simulink model "soc_dvbs2_fpga"  (R2025b)
settings: Solver=FixedStepDiscrete  StartTime=0.0  StopTime=0  RelTol=1e-3
InitFcn:
  | soc_dvbs2_init;
values from neighbouring files (symbols this model uses):
  Rsym = 4e6    (= 4000000)    [soc_dvbs2_init.m]
  soc_dvbs2_txPacketBits = [1 1 0 1 0 1 1 1 0 1 1 1 ... (2972 elements, 2972x1)]    [soc_dvbs2_txPacketBits.mat]
  syncWord = (dec2bin(hex2dec('AC')) - '0').'    [soc_dvbs2_init.m]
  txDataOut = txobj(frameBits(:))    [soc_dvbs2_init.m]
  txFiltCoeff = txobj.pTxFilterCoeff    [soc_dvbs2_init.m]
undefined symbols (not defined in the file or in its folder): Add, coefficientsLog, coefficientsSqrt1, coefficientsSqrt2, dataBits, designMultirateFIR, noisePow, NumBits1, NumBits2, seedsURNG1, seedsURNG2, Shift, Slope1, Slope2, soc_dvbs2_designFIRFilter, txDataOutS1, txDataOutS10, txDataOutS12, txDataOutS13, txDataOutS14, txDataOutS15, txDataOutS16, txDataOutS18, txDataOutS19, txDataOutS2, txDataOutS20, txDataOutS21, txDataOutS22, txDataOutS24, txDataOutS25, txDataOutS26, txDataOutS27, txDataOutS3, txDataOutS4, txDataOutS5, txDataOutS6, txDataOutS7, txDataOutS8, txDataOutS9
libraries: simulink x214, hdlsllib x211, dspsigops x22, dsphdlfiltering2 x8, dsphdlsigops2 x5, commseqgen3 x5, dsphdlmathfun2 x3, hwlogicconnlib x2, whdledac x2, commhdlcrc x2, whdlutilities x1, whdlmod x1
(part 8 of 12)

== system soc_dvbs2_fpga/DVBS2/DVBS2 TxRx/DVB-S2 HDL Receiver/Synchronizer and PL Header Decoder/Time Frequency and Coarse Phase Synchronizer/Fine Frequency Synchronizer/Modified L and R Algorithm/L and R Algorithm 18 point ==
  z : Inport
  zvalid : Inport  Port=2
  Add : Sum  Inputs=+++
  Compute R(m) for 1 to 6 : Subsystem  mask{m=1:6}
      mask prompts: m "m values for computing R(m):"
  Compute R(m) for 13 to 18 : Subsystem  mask{m=13:18}
      mask prompts: m "m values for computing R(m):"
  Compute R(m) for 7 to 12 : Subsystem  mask{m=7:12}
      mask prompts: m "m values for computing R(m):"
  Data Type Conversion : DataTypeConversion  OutDataTypeStr=fixdt(1,16,11)  SaturateOnIntegerOverflow=off  RndMeth=Floor
  Delay{1..6} (6 alike) : Delay
  dataIn : Outport
  wires:
  Data Type Conversion/1 -> Delay3/1
  Add/1 -> Delay6/1
  z/1 -> Data Type Conversion/1
  Delay3/1 -> Compute R(m) for 1 to 6/1(z), Compute R(m) for 13 to 18/1(z), Compute R(m) for 7 to 12/1(z)
  Delay2/1 -> Add/1
  Delay6/1 -> dataIn/1
  Delay5/1 -> Add/3
  Delay4/1 -> Add/2
  Delay1/1 -> Compute R(m) for 1 to 6/2(zvalid), Compute R(m) for 13 to 18/2(zvalid), Compute R(m) for 7 to 12/2(zvalid)
  Compute R(m) for 13 to 18/1(sum) -> Delay5/1
  Compute R(m) for 7 to 12/1(sum) -> Delay4/1
  Compute R(m) for 1 to 6/1(sum) -> Delay2/1
  zvalid/1 -> Delay1/1

== system soc_dvbs2_fpga/DVBS2/DVBS2 TxRx/DVB-S2 HDL Receiver/Synchronizer and PL Header Decoder/Time Frequency and Coarse Phase Synchronizer/Fine Frequency Synchronizer/Modified L and R Algorithm/Moving Average ==
  dataIn : Inport
  validIn : Inport  Port=2
  Add : Sum  Inputs=|++  OutDataTypeStr=Inherit: Inherit via back propagation
  Add1 : Sum  Inputs=|+-
  Data Type Duplicate : DataTypeDuplicate
  Data Type Conversion1 : DataTypeConversion  OutDataTypeStr=fixdt(1,53,36)  SaturateOnIntegerOverflow=off  RndMeth=Floor
  Delay : Delay  DelayLength=config.FFCAveragingLength  ShowEnablePort=on
      settings: InputPortMap=u0,e6
  Delay1 : Delay  DelayLength=1  ShowEnablePort=on
      settings: InputPortMap=u0,e6
  Delay2 : Delay
  Delay3 : Delay
  Delay{4..8} (5 alike) : Delay  DelayLength=1
  Gain : Gain  Gain=1/config.FFCAveragingLength  ParamDataTypeStr=fixdt(0,nextpow2(config.FFCAveragingLength),nextpow2(config.FFCAveragingLength))  OutDataTypeStr=Inherit: Same as input
  dataOut : Outport
  validOut : Outport  Port=2
  wires:
  Data Type Conversion1/1 -> Delay3/1
  Delay8/1 -> validOut/1
  Delay4/1 -> dataOut/1
  Gain/1 -> Add/1, Data Type Duplicate/1
  Delay7/1 -> Delay2/1
  Delay6/1 -> Add1/2
  Delay5/1 -> Add1/1
  Delay2/1 -> Delay1/2, Delay8/1
  Delay3/1 -> Gain/1
  validIn/1 -> Delay/2, Delay7/1
  Delay/1 -> Delay6/1
  Add1/1 -> Data Type Conversion1/1
  Add/1 -> Delay1/1, Delay4/1, Data Type Duplicate/2
  Delay1/1 -> Add/2
  dataIn/1 -> Delay/1, Delay5/1

== system soc_dvbs2_fpga/DVBS2/DVBS2 TxRx/DVB-S2 HDL Receiver/Synchronizer and PL Header Decoder/Time Frequency and Coarse Phase Synchronizer/Fine Gain Control/Reciprocal/Function Impl ==
  switch : Inport
  LUTAddr : Inport  Port=2
  Delay{6..8,10,15..16} (6 alike) : Delay
  Delay9 : Delay  DelayLength=1
  LUT1 : LookupNDDirect  NumberOfTableDimensions=1  Table=LUT(:,1)  DiagnosticForOutOfRangeInput=Error
  LUT2 : LookupNDDirect  NumberOfTableDimensions=1  Table=LUT(:,2)  DiagnosticForOutOfRangeInput=Error
  Multiport Switch : MultiPortSwitch  DataPortOrder=Zero-based contiguous  Inputs=2  zeroidx=on  SaturateOnIntegerOverflow=off  InputSameDT=off
  functionValues : Outport
  wires:
  LUTAddr/1 -> Delay7/1, Delay6/1
  Delay15/1 -> Multiport Switch/2
  Delay16/1 -> Multiport Switch/3
  Delay10/1 -> Multiport Switch/1
  Delay9/1 -> functionValues/1
  LUT2/1 -> Delay15/1
  LUT1/1 -> Delay16/1
  switch/1 -> Delay8/1
  Delay8/1 -> Delay10/1
  Delay7/1 -> LUT2/1
  Delay6/1 -> LUT1/1
  Multiport Switch/1 -> Delay9/1

== system soc_dvbs2_fpga/DVBS2/DVBS2 TxRx/DVB-S2 HDL Receiver/Synchronizer and PL Header Decoder/Time Frequency and Coarse Phase Synchronizer/Time and Coarse Frequency Synchronizer/Coarse Frequency Estimator/Direct Digital Synthesis ==
  v : Inport
  rst : Inport  Port=2
  Constant : Constant  Value=true  SampleTime=-1
  Data Type Conversion : DataTypeConversion  OutDataTypeStr=fixdt(1,21,21)  SaturateOnIntegerOverflow=off  RndMeth=Floor
  Data Type Conversion1 : DataTypeConversion  OutDataTypeStr=fixdt(1,21,0)  ConvertRealWorld=Stored Integer (SI)  SaturateOnIntegerOverflow=off  RndMeth=Floor
  Delay1 : Delay
  Delay14 : Delay
  Delay2 : Delay  DelayLength=1  InitialCondition=0
  Gain : Gain  Gain=1/config.SamplesPerSymbol  ParamDataTypeStr=fixdt(0,2,2)  OutDataTypeStr=Inherit: Same as input
  NCO HDL Optimized : dsphdlsigops2/NCO  PhaseIncrementSource=Input port  PhaseIncrement=100  PhaseOffsetSource=Property  PhaseOffset=0  DitherSource=None  NumDitherBits=11  SamplesPerFrame=1  LUTCompress=off  ResetAction=on  Waveform=Complex exponential  PhasePort=off  SimulateUsing=Code generation  AccumulatorWL=21  PhaseQuantization=on  NumQuantizerAccumulatorBits=14  OutputDataType=Binary point scaling  OutputWL=16  OutputFL=14
  Repeat : dspsigops/Repeat  FactorSource=Dialog parameter  N=config.SamplesPerSymbol  Nmax=16  RateOptions=Allow multirate processing  ic=0  mode=Unused parameter value
  Repeat1 : dspsigops/Repeat  FactorSource=Dialog parameter  N=config.SamplesPerSymbol  Nmax=16  RateOptions=Allow multirate processing  ic=0  mode=Unused parameter value
  Terminator : Terminator
  complexEst : Outport
  normalizedEst : Outport  Port=2
  wires:
  Repeat1/1 -> NCO HDL Optimized/2
  rst/1 -> Repeat1/1
  Data Type Conversion/1 -> normalizedEst/1, Data Type Conversion1/1
  Repeat/1 -> NCO HDL Optimized/1
  Constant/1 -> NCO HDL Optimized/3
  Data Type Conversion1/1 -> Repeat/1
  Delay2/1 -> complexEst/1
  Delay1/1 -> Data Type Conversion/1
  Delay14/1 -> Gain/1
  NCO HDL Optimized/1 -> Delay2/1
  v/1 -> Delay14/1
  NCO HDL Optimized/2 -> Terminator/1
  Gain/1 -> Delay1/1

== system soc_dvbs2_fpga/DVBS2/DVBS2 TxRx/DVB-S2 HDL Receiver/Synchronizer and PL Header Decoder/Time Frequency and Coarse Phase Synchronizer/Time and Coarse Frequency Synchronizer/Coarse Frequency Estimator/Frequency Error Detector ==
  dataIn : Inport
  pilotIdx : Inport  Port=2
  pilotValid : Inport  Port=3
  Compare To Constant1 : simulink/Logic and Bit Operations/Compare To Constant  relop=<=  const=config.PilotMaxIdx - 2  OutDataTypeStr=boolean
  Compare To Constant2 : simulink/Logic and Bit Operations/Compare To Constant  relop=>=  const=config.PilotMinIdx + 2  OutDataTypeStr=boolean
  Complex Multiplier : Subsystem  VariantControl=Use 3 multipliers and 5 adders
      mask Display: disp(['Complex Multiplier' newline 'Latency = 8']);
  Complex to Real-Imag : ComplexToRealImag  Output=Imag
  Delay{,1..11,16..19,24} (17 alike) : Delay
  Delay12 : Delay  DelayLength=1
  Delay13 : Delay  DelayLength=1
  Delay14 : Delay  DelayLength=1
  Delay15 : Delay  DelayLength=8
  Gain : Gain  Gain=conj(config.Pilot)  OutDataTypeStr=Inherit: Same as input
      mask init:
      | Simulink.suppressDiagnostic(gcb, 'SimulinkFixedPoint:util:fxpParameterPrecisionLoss');
  Gain1 : Gain  Gain=config.Pilot  OutDataTypeStr=Inherit: Same as input
      mask init:
      | Simulink.suppressDiagnostic(gcb, 'SimulinkFixedPoint:util:fxpParameterPrecisionLoss');
  Logical Operator : Logic  Inputs=3  AllPortsSameDT=off  OutDataTypeStr=boolean
  Math Function : Math  Operator=conj
  Unit Delay Enabled Synchronous : hdlsllib/Discrete/Unit Delay Enabled Synchronous  InitialCondition=0.0  SampleTime=-1
  e : Outport
  wires:
  Delay19/1 -> Complex Multiplier/1(In1)
  Delay17/1 -> Complex Multiplier/2(In2)
  Delay16/1 -> Delay15/1
  Delay14/1 -> e/1
  Complex Multiplier/1(Out1) -> Delay10/1
  Delay18/1 -> Logical Operator/2
  Compare To Constant1/1 -> Delay18/1
  Logical Operator/1 -> Delay8/1
  Gain1/1 -> Delay6/1
  Gain/1 -> Delay4/1
  Delay15/1 -> Delay11/1
  Delay7/1 -> Delay17/1
  Delay5/1 -> Delay19/1
  Delay13/1 -> Unit Delay Enabled Synchronous/2
  Delay12/1 -> Unit Delay Enabled Synchronous/1
  Delay11/1 -> Delay13/1
  Delay10/1 -> Complex to Real-Imag/1
  Delay9/1 -> Delay16/1
  Delay8/1 -> Delay9/1
  Delay6/1 -> Delay7/1
  Delay4/1 -> Delay5/1
  Delay3/1 -> Logical Operator/3
  Delay2/1 -> Logical Operator/1
  Delay1/1 -> Gain1/1
  Delay24/1 -> Gain/1
  Complex to Real-Imag/1 -> Delay12/1
  pilotValid/1 -> Delay3/1
  Compare To Constant2/1 -> Delay2/1
  pilotIdx/1 -> Compare To Constant2/1, Compare To Constant1/1
  Unit Delay Enabled Synchronous/1 -> Delay14/1
  Math Function/1 -> Delay1/1
  dataIn/1 -> Delay/1, Delay24/1
  Delay/1 -> Math Function/1

== system soc_dvbs2_fpga/DVBS2/DVBS2 TxRx/DVB-S2 HDL Receiver/Synchronizer and PL Header Decoder/Time Frequency and Coarse Phase Synchronizer/Time and Coarse Frequency Synchronizer/Coarse Frequency Estimator/Loop Filter ==
  e : Inport
  rst : Inport  Port=2
  En : Inport  Port=3
  Add : Sum  Inputs=|++  OutDataTypeStr=Inherit: Same as first input
  Delay{,1..3} (4 alike) : Delay  DelayLength=1
  Delay14 : Delay
  Integrator Gain : Gain  Gain=fi(config.CFCLoopFilterIntegGain/(2*pi),0,16)  ParamDataTypeStr=Inherit: Inherit from 'Gain'  OutDataTypeStr=Inherit: Same as input
  Unit Delay Enabled Resettable Synchronous : hdlsllib/Discrete/Unit Delay Enabled Resettable Synchronous  InitialCondition=0.0  SampleTime=-1
  v : Outport
  rstOut : Outport  Port=2
  wires:
  Delay/1 -> Delay3/1
  Delay3/1 -> rstOut/1
  rst/1 -> Unit Delay Enabled Resettable Synchronous/3, Delay/1
  Add/1 -> Unit Delay Enabled Resettable Synchronous/1
  En/1 -> Unit Delay Enabled Resettable Synchronous/2
  Unit Delay Enabled Resettable Synchronous/1 -> Delay2/1, Add/2
  Delay1/1 -> Add/1
  Delay2/1 -> v/1
  Delay14/1 -> Integrator Gain/1
  e/1 -> Delay14/1
  Integrator Gain/1 -> Delay1/1

== system soc_dvbs2_fpga/DVBS2/DVBS2 TxRx/DVB-S2 HDL Receiver/Synchronizer and PL Header Decoder/Time Frequency and Coarse Phase Synchronizer/Time and Coarse Frequency Synchronizer/Coarse Frequency Estimator/Pilot Blks Counter ==
  pilotIdx : Inport
  pilotValid : Inport  Port=2
  rst : Inport  Port=3
  Compare To Constant : simulink/Logic and Bit Operations/Compare To Constant  relop===  const=config.PilotMinIdx  OutDataTypeStr=boolean
  HDL Counter : hdlsllib/Sources/HDL Counter  CountType=Free running  CountInit=0  CountStep=1  CountMax=25  CountFromType=Initial value  CountFrom=0  CountResetPort=on  CountLoadPort=off  CountEnbPort=on  CountDirPort=off  CountHitOutputPort=off  CountDataType=Unsigned  CountWordLen=16  CountFracLen=0  CountSampTime=1
  Logical Operator : Logic  AllPortsSameDT=off  OutDataTypeStr=boolean
  pilotBlkCount : Outport
  wires:
  rst/1 -> HDL Counter/1
  HDL Counter/1 -> pilotBlkCount/1
  pilotIdx/1 -> Compare To Constant/1
  pilotValid/1 -> Logical Operator/2
  Compare To Constant/1 -> Logical Operator/1
  Logical Operator/1 -> HDL Counter/2

== system soc_dvbs2_fpga/DVBS2/DVBS2 TxRx/DVB-S2 HDL Receiver/Synchronizer and PL Header Decoder/Time Frequency and Coarse Phase Synchronizer/Time and Coarse Frequency Synchronizer/Frame Synchronizer/Correlator ==
  note: Differential Detection
  note: Compute Energy
  dataIn : Inport
  validIn : Inport  Port=2
  Add4 : Sum
  Complex to Real-Imag : ComplexToRealImag  Output=Real
  Data Type Conversion : DataTypeConversion  OutDataTypeStr=fixdt(1,17,14)  SaturateOnIntegerOverflow=off  RndMeth=Floor
  Delay{,9..10,12} (4 alike) : Delay  DelayLength=1
  Delay{1..2,4..8,11,13..25} (21 alike) : Delay
  Delay3 : Delay  DelayLength=70-32
  Gain : Gain  Gain=fi(config.refSOFE,0,16,16)  OutDataTypeStr=fixdt(1,32,30)
  Gain1 : Gain  Gain=fi(config.refPLSCE,0,16,16)  OutDataTypeStr=fixdt(1,32,30)
  Math Function : Math  Operator=conj
  Math Function1 : Math  Operator=conj
  Moving Sum : Subsystem
  PLSC Correlator : Subsystem  mask{coefs=config.refPLSC, shareFactor=4}
      mask prompts: coefs "Coefficients:"; shareFactor "Number of cycles:"
      mask init:
      | ob                         = dsphdl.FIRFilter('Numerator',coefs);
      | directFormLatency          = getLatency(ob);
      | 
      | ob                         = dsphdl.FIRFilter('Numerator',coefs,...
      |                                               'FilterStructure','Partly Serial Systolic',...
      |                                               'NumCycles',shareFactor);
      | partlySerialLatency        = getLatency(ob);
      | partlySerialExtraDelay     = 4 - mod(partlySerialLatency,4);
      | 
      | adjustDelay                = directFormLatency - ...
      |                             (partlySerialLatency+partlySerialExtraDelay)/shareFactor;
  Product : Product  OutDataTypeStr=Inherit: Same as first input
  Product1 : Product  OutDataTypeStr=Inherit: Same as first input
  SOF Correlator : Subsystem  mask{coefs=config.refSOF, shareFactor=4}
      mask prompts: coefs "Coefficients:"; shareFactor "Number of cycles:"
      mask init: same as soc_dvbs2_fpga/DVBS2/DVBS2 TxRx/DVB-S2 HDL Receiver/Synchronizer and PL Header Decoder/Time Frequency and Coarse Phase Synchronizer/Time and Coarse Frequency Synchronizer/Frame Synchronizer/Correlator/PLSC Correlator
  SOFCorrOut : Outport
  PLSCCorrOut : Outport  Port=2
  threshold : Outport  Port=3
  wires:
  SOF Correlator/1(dataOut) -> Delay3/1
  Delay25/1 -> Moving Sum/3(validIn)
  Delay11/1 -> Delay25/1
  Delay24/1 -> Delay4/1
  Delay23/1 -> Delay5/1
  Delay22/1 -> Delay6/1
  Delay21/1 -> Delay11/1
  Delay20/1 -> Complex to Real-Imag/1
  Delay19/1 -> Product1/1
  Delay18/1 -> Product1/2
  Delay17/1 -> Delay21/1
  Delay16/1 -> Gain1/1
  Delay15/1 -> Gain/1
  Delay14/1 -> Moving Sum/1(scaled1)
  Delay13/1 -> Moving Sum/2(scaled2)
  dataIn/1 -> Delay1/1, Delay19/1, Math Function1/1
  Math Function1/1 -> Delay18/1
  Complex to Real-Imag/1 -> Delay16/1, Delay15/1
  Add4/1 -> Delay12/1
  Delay12/1 -> Data Type Conversion/1
  Product1/1 -> Delay20/1
  Gain/1 -> Delay14/1
  validIn/1 -> Delay17/1, Delay2/1
  Gain1/1 -> Delay13/1
  Moving Sum/1(E1) -> Add4/1
  Moving Sum/2(E2) -> Add4/2
  PLSC Correlator/1(dataOut) -> Delay10/1
  Delay3/1 -> Delay9/1
  Product/1 -> Delay7/1
  Math Function/1 -> Delay24/1
  Delay/1 -> Delay23/1
  Delay1/1 -> Math Function/1, Delay/1
  Delay2/1 -> Delay22/1
  Delay4/1 -> Product/1
  Delay5/1 -> Product/2
  Delay6/1 -> Delay8/1
  Delay8/1 -> SOF Correlator/2(validIn), PLSC Correlator/2(validIn)
  Delay7/1 -> SOF Correlator/1(dataIn), PLSC Correlator/1(dataIn)
  Delay10/1 -> PLSCCorrOut/1
  Delay9/1 -> SOFCorrOut/1
  Data Type Conversion/1 -> threshold/1

== system soc_dvbs2_fpga/DVBS2/DVBS2 TxRx/DVB-S2 HDL Receiver/Synchronizer and PL Header Decoder/Time Frequency and Coarse Phase Synchronizer/Time and Coarse Frequency Synchronizer/Frame Synchronizer/Pilot and Sync Pulse Indicator ==
  note: Compute Energy
  note: Compute Energy
  SOFCorrDelayed : Inport
  PLSCCorr : Inport  Port=2
  threshold : Inport  Port=3
  Bus Creator : BusCreator  Inputs=3
  Complex to Real-Imag : ComplexToRealImag  Output=Real
  Complex to Real-Imag1 : ComplexToRealImag  Output=Real
  Corr Add : Sum
  Corr Subtract : Sum  Inputs=+-
  Delay{1..10,15..16,19..21,24..26} (18 alike) : Delay  DelayLength=1
  Delay{11..14,17..18,22..23} (8 alike) : Delay
  Logical Operator : Logic  Operator=OR  AllPortsSameDT=off  OutDataTypeStr=boolean
  Math Function : Math  Operator=conj
  Math Function1 : Math  Operator=conj
  No HDL Correlation Value : Subsystem
  Product : Product  OutDataTypeStr=fixdt(1,18,15)
  Product1 : Product  OutDataTypeStr=fixdt(1,18,15)
  Relational Operator : RelationalOperator  Operator=>  OutDataTypeStr=boolean  RndMeth=Simplest  InputSameDT=off
  Relational Operator1 : RelationalOperator  Operator=>  OutDataTypeStr=boolean  RndMeth=Simplest  InputSameDT=off
  Threshold Scaling : Gain  Gain=config.Threshold  OutDataTypeStr=Inherit: Same as input
      mask init:
      | Simulink.suppressDiagnostic(gcb, 'SimulinkFixedPoint:util:fxpParameterPrecisionLoss');
  ThresholdLimiter : MATLAB Function  TreatAsAtomicUnit=on
  hasPilots : Outport
  thresholdExceeded : Outport  Port=2
  VisualizeCorrelationSignals : Outport  Port=3
  wires:
  Delay9/1 -> hasPilots/1, No HDL Correlation Value/2(In1)
  Complex to Real-Imag1/1 -> Delay1/1
  Complex to Real-Imag/1 -> Delay6/1
  Delay24/1 -> Delay22/1
  Delay12/1 -> Complex to Real-Imag1/1
  Delay19/1 -> Math Function1/1
  Delay18/1 -> Product1/2
  Delay20/1 -> Delay17/1
  Delay17/1 -> Product1/1
  Corr Subtract/1 -> Delay20/1, Delay19/1
  Product1/1 -> Delay12/1
  Math Function1/1 -> Delay18/1
  ThresholdLimiter/1(y) -> Delay26/1
  Delay10/1 -> thresholdExceeded/1
  Delay25/1 -> ThresholdLimiter/1(x)
  Delay23/1 -> Delay25/1
  Threshold Scaling/1 -> Delay23/1
  Delay22/1 -> Threshold Scaling/1
  Delay21/1 -> Delay24/1
  threshold/1 -> Delay21/1
  PLSCCorr/1 -> Delay5/1, Delay3/1
  SOFCorrDelayed/1 -> Delay4/1, Delay2/1
  Delay1/1 -> Delay8/1
  Delay6/1 -> Delay7/1
  Product/1 -> Delay11/1
  Delay16/1 -> Delay13/1
  Delay15/1 -> Math Function/1
  Delay14/1 -> Product/2
  Delay11/1 -> Complex to Real-Imag/1
  Math Function/1 -> Delay14/1
  Corr Add/1 -> Delay16/1, Delay15/1
  Delay13/1 -> Product/1
  Delay5/1 -> Corr Subtract/2
  Delay4/1 -> Corr Subtract/1
  Delay3/1 -> Corr Add/2
  Delay2/1 -> Corr Add/1
  Relational Operator/1 -> Logical Operator/1, Delay9/1
  Logical Operator/1 -> Delay10/1
  Relational Operator1/1 -> Logical Operator/2
  Delay7/1 -> Bus Creator/1, No HDL Correlation Value/1(PeakValueWithPilots), Relational Operator/1  "PeakValueWithPilots"
  Delay26/1 -> Relational Operator/2, Bus Creator/3, Relational Operator1/2  "Threshold"
  Delay8/1 -> Bus Creator/2, No HDL Correlation Value/3(PeakValueWithoutPilots), Relational Operator1/1  "PeakValueWithoutPilots"
  Bus Creator/1 -> VisualizeCorrelationSignals/1  "VisualizeCorrelationSignals"

== system soc_dvbs2_fpga/DVBS2/DVBS2 TxRx/DVB-S2 HDL Receiver/Synchronizer and PL Header Decoder/Time Frequency and Coarse Phase Synchronizer/Time and Coarse Frequency Synchronizer/PL Data Descrambler and Pilot Valid Indicator/PL Data Descrambler ==
  reset : Inport
  inputCount : Inport  Port=2
  validIn : Inport  Port=3
  dataIn : Inport  Port=4
  Compare To Constant : simulink/Logic and Bit Operations/Compare To Constant  relop=<=  const=config.PLSCLength - 1  OutDataTypeStr=boolean
  Delay1 : Delay  DelayLength=7
  Delay{2..8,10..12,22..23} (12 alike) : Delay  DelayLength=1
  Delay{13..21} (9 alike) : Delay
  Delay9 : Delay  DelayLength=7
  Math Function : Math  Operator=conj
  PL Scramble Sequence Mapper LUT : Lookup_n-D  NumberOfTableDimensions=1  LookupTableObject=''  BreakpointsSpecification=Even spacing  BreakpointsForDimension1=[-5:5]  BreakpointsForDimension1FirstPoint=0  BreakpointsForDimension2FirstPoint=10  BreakpointsForDimension2Spacing=12  IndexSearchMethod=Evenly spaced points  Table=[1;1i;-1;-1i]  TableDataTypeStr=fixdt(1,2,0)  InterpMethod=Flat  DiagnosticForOutOfRangeInput=Error  InternalRulePriority=Speed  OutDataTypeStr=fixdt(1,2,0)  RndMeth=Simplest
  PL Scrambler Gold Sequence Generator : Subsystem  mask{n=0}
      mask prompts: n "Index of Gold Sequence :"
  Product : Product  OutDataTypeStr=Inherit: Same as first input
  Switch : Switch  Criteria=u2 ~= 0  SaturateOnIntegerOverflow=off  InputSameDT=off
  dataOut : Outport
  validOut : Outport  Port=2
  wires:
  Delay12/1 -> Delay13/1
  Delay23/1 -> validOut/1
  Delay22/1 -> dataOut/1
  Delay21/1 -> Delay23/1
  Delay20/1 -> Switch/3
  Delay19/1 -> Switch/2
  Delay18/1 -> Switch/1
  Delay17/1 -> Delay21/1
  Delay16/1 -> Product/2
  Delay15/1 -> Product/1
  Delay14/1 -> Delay19/1
  Delay13/1 -> Delay18/1
  Delay11/1 -> Compare To Constant/1
  Delay10/1 -> Delay15/1
  Delay8/1 -> Delay17/1
  Delay7/1 -> Math Function/1
  Delay6/1 -> Delay12/1
  Delay5/1 -> Delay8/1
  Delay4/1 -> Delay10/1
  Delay3/1 -> Delay11/1
  Delay2/1 -> PL Scramble Sequence Mapper LUT/1
  Delay1/1 -> Delay3/1
  Delay9/1 -> Delay6/1, Delay4/1
  validIn/1 -> PL Scrambler Gold Sequence Generator/2(validIn)
  reset/1 -> PL Scrambler Gold Sequence Generator/1(reset)
  PL Scrambler Gold Sequence Generator/2(validOut) -> Delay5/1
  Switch/1 -> Delay22/1
  Product/1 -> Delay20/1
  PL Scramble Sequence Mapper LUT/1 -> Delay7/1
  dataIn/1 -> Delay9/1
  Math Function/1 -> Delay16/1
  inputCount/1 -> Delay1/1
  Compare To Constant/1 -> Delay14/1
  PL Scrambler Gold Sequence Generator/1(dataOut) -> Delay2/1

== system soc_dvbs2_fpga/DVBS2/DVBS2 TxRx/DVB-S2 HDL Receiver/Synchronizer and PL Header Decoder/Time Frequency and Coarse Phase Synchronizer/Time and Coarse Frequency Synchronizer/PL Data Descrambler and Pilot Valid Indicator/Pilot Valid Indicator ==
  note: Hold pilotEnable signal
  note: Hold pilotsEnable signal after endOfPLSC
  pilotEnable : Inport
  validIn : Inport  Port=2
  endOfSOFIn : Inport  Port=3
  endOfPLSC : Inport  Port=4
  Compare To Constant2 : simulink/Logic and Bit Operations/Compare To Constant  relop=>=  const=config.PilotMinIdx  OutDataTypeStr=boolean
  Compare To Constant3 : simulink/Logic and Bit Operations/Compare To Constant  relop=<=  const=config.PilotMaxIdx  OutDataTypeStr=boolean
  Delay{1..4} (4 alike) : Delay  DelayLength=config.SOFLength
  Delay{5..14,19} (11 alike) : Delay  DelayLength=1
  Delay15 : Delay
  Delay16 : Delay
  Delay17 : Delay
  Logical Operator1 : Logic  Inputs=3  AllPortsSameDT=off  OutDataTypeStr=boolean
  Logical Operator2 : Logic  AllPortsSameDT=off  OutDataTypeStr=boolean
  Logical Operator3 : Logic  AllPortsSameDT=off  OutDataTypeStr=boolean
  PilotIdx Counter : hdlsllib/Sources/HDL Counter  CountType=Count limited  CountInit=0  CountStep=1  CountMax=config.PilotMaxIdx  CountFromType=Initial value  CountFrom=0  CountResetPort=on  CountLoadPort=off  CountEnbPort=on  CountDirPort=off  CountHitOutputPort=off  CountDataType=Unsigned  CountWordLen=nextpow2(config.PilotMaxIdx)  CountFracLen=0  CountSampTime=1
  Unit Delay Enabled Resettable Synchronous : hdlsllib/Discrete/Unit Delay Enabled Resettable Synchronous  InitialCondition=0.0  SampleTime=-1
  Unit Delay Enabled Resettable Synchronous1 : hdlsllib/Discrete/Unit Delay Enabled Resettable Synchronous  InitialCondition=0.0  SampleTime=-1
  pilotValid : Outport
  pilotIdx : Outport  Port=2
  endOfSOF : Outport  Port=3
  wires:
  Delay17/1 -> endOfSOF/1
  Delay16/1 -> pilotValid/1
  Delay15/1 -> pilotIdx/1
  Delay14/1 -> Delay17/1
  Delay13/1 -> Logical Operator1/3
  Delay12/1 -> Logical Operator1/2
  Delay11/1 -> Logical Operator1/1
  Delay10/1 -> Delay15/1
  Delay9/1 -> Delay14/1
  Delay8/1 -> Delay13/1
  Delay7/1 -> Logical Operator3/2
  Delay6/1 -> Compare To Constant3/1
  Delay5/1 -> Compare To Constant2/1
  Delay19/1 -> Delay10/1
  Logical Operator3/1 -> Delay12/1
  Unit Delay Enabled Resettable Synchronous/1 -> Logical Operator2/2
  Unit Delay Enabled Resettable Synchronous1/1 -> Delay8/1
  Delay2/1 -> Delay9/1, Unit Delay Enabled Resettable Synchronous/2
  Delay1/1 -> Unit Delay Enabled Resettable Synchronous/1
  Delay4/1 -> Delay7/1, PilotIdx Counter/2
  Delay3/1 -> Logical Operator2/1, PilotIdx Counter/1
  endOfSOFIn/1 -> Delay2/1, Unit Delay Enabled Resettable Synchronous/3, Unit Delay Enabled Resettable Synchronous1/3
  pilotEnable/1 -> Delay1/1
  Logical Operator1/1 -> Delay16/1
  Logical Operator2/1 -> Unit Delay Enabled Resettable Synchronous1/2, Unit Delay Enabled Resettable Synchronous1/1
  validIn/1 -> Delay4/1
  Compare To Constant2/1 -> Delay11/1
  PilotIdx Counter/1 -> Delay19/1, Delay5/1, Delay6/1
  endOfPLSC/1 -> Delay3/1
  Compare To Constant3/1 -> Logical Operator3/1

== system soc_dvbs2_fpga/DVBS2/DVBS2 TxRx/DVB-S2 HDL Receiver/Synchronizer and PL Header Decoder/Time Frequency and Coarse Phase Synchronizer/Time and Coarse Frequency Synchronizer/Symbol Synchronizer/Gardner TED ==
  data : Inport
  strobe : Inport  Port=2
  Constant : Constant  Value=0  OutDataTypeStr=Inherit: Inherit via back propagation  SampleTime=-1
  Delay10 : Delay  DelayLength=4
  GTED : Subsystem
  Switch : Switch  Criteria=u2 ~= 0  InputSameDT=off
  e : Outport  VectorParamsAs1DForOutWhenUnconnected=off
  wires:
  Delay10/1 -> Switch/2
  GTED/1(Out1) -> Switch/1
  data/1 -> GTED/1(In1)
  strobe/1 -> Delay10/1
  Switch/1 -> e/1
  Constant/1 -> Switch/3

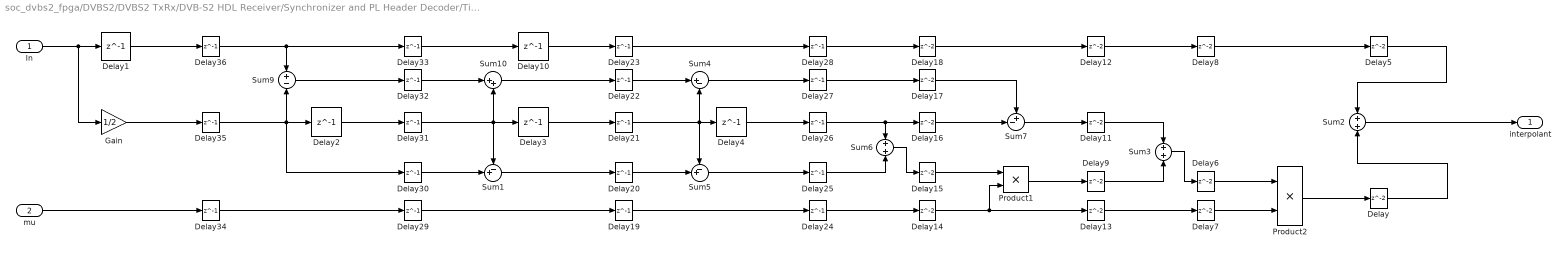
== system soc_dvbs2_fpga/DVBS2/DVBS2 TxRx/DVB-S2 HDL Receiver/Synchronizer and PL Header Decoder/Time Frequency and Coarse Phase Synchronizer/Time and Coarse Frequency Synchronizer/Symbol Synchronizer/Interpolation Filter ==
  In : Inport
  mu : Inport  Port=2
  Delay{,5..9,11..18} (14 alike) : Delay
  Delay{1..4,10} (5 alike) : Delay  DelayLength=1  InitialCondition=0
  Delay{19..36} (18 alike) : Delay  DelayLength=1
  Gain : Gain  Gain=1/2  ParamDataTypeStr=fixdt(0,1,1)  OutDataTypeStr=Inherit: Same as input
  Product1 : Product  RndMeth=Zero  OutDataTypeStr=Inherit: Same as first input
  Product2 : Product  RndMeth=Zero  OutDataTypeStr=Inherit: Same as first input
  Sum1 : Sum  Inputs=-+|
  Sum10 : Sum  Inputs=|++
  Sum2 : Sum  Inputs=+|+
  Sum3 : Sum  Inputs=+|+  OutDataTypeStr=Inherit: Same as first input
  Sum4 : Sum  Inputs=|+-
  Sum5 : Sum  Inputs=-+|
  Sum6 : Sum  Inputs=+|+  SaturateOnIntegerOverflow=on  OutDataTypeStr=Inherit: Same as first input
  Sum7 : Sum  Inputs=+-|  OutDataTypeStr=Inherit: Same as first input
  Sum9 : Sum  Inputs=+-
  interpolant : Outport
  wires:
  Delay36/1 -> Sum9/1, Delay33/1
  Delay35/1 -> Sum9/2, Delay2/1, Delay30/1
  Delay34/1 -> Delay29/1
  Delay33/1 -> Delay10/1
  Delay32/1 -> Sum10/1
  Delay31/1 -> Delay3/1, Sum10/2, Sum1/1
  Delay30/1 -> Sum1/2
  Delay29/1 -> Delay19/1
  Delay23/1 -> Delay28/1
  Delay22/1 -> Sum4/1
  Delay21/1 -> Delay4/1, Sum5/1, Sum4/2
  Delay20/1 -> Sum5/2
  Delay19/1 -> Delay24/1
  Delay25/1 -> Sum6/2
  Delay28/1 -> Delay18/1
  Delay27/1 -> Delay17/1
  Delay26/1 -> Sum6/1, Delay16/1
  Sum6/1 -> Delay15/1
  Delay24/1 -> Delay14/1
  Delay10/1 -> Delay23/1
  Sum4/1 -> Delay27/1
  Delay4/1 -> Delay26/1
  Sum5/1 -> Delay25/1
  mu/1 -> Delay34/1
  Delay18/1 -> Delay12/1
  Delay17/1 -> Sum7/1
  Delay16/1 -> Sum7/2
  Delay15/1 -> Product1/1
  Delay14/1 -> Product1/2, Delay13/1
  Delay13/1 -> Delay7/1
  Delay12/1 -> Delay8/1
  Delay11/1 -> Sum3/1
  Delay9/1 -> Sum3/2
  Delay8/1 -> Delay5/1
  Delay7/1 -> Product2/2
  Delay6/1 -> Product2/1
  Delay5/1 -> Sum2/1
  Delay/1 -> Sum2/2
  Gain/1 -> Delay35/1
  Delay1/1 -> Delay36/1
  Delay2/1 -> Delay31/1
  Sum10/1 -> Delay22/1
  Delay3/1 -> Delay21/1
  Sum1/1 -> Delay20/1
  Sum3/1 -> Delay6/1
  Product2/1 -> Delay/1
  Product1/1 -> Delay9/1
  Sum7/1 -> Delay11/1
  Sum2/1 -> interpolant/1
  In/1 -> Gain/1, Delay1/1
  Sum9/1 -> Delay32/1

== system soc_dvbs2_fpga/DVBS2/DVBS2 TxRx/DVB-S2 HDL Receiver/Synchronizer and PL Header Decoder/Time Frequency and Coarse Phase Synchronizer/Time and Coarse Frequency Synchronizer/Symbol Synchronizer/Loop Filter ==
  note: Proportional-Plus-Integrator Loop Filter,
      | Infinite DC Response to guarantee convergence
  e : Inport
  Add : Sum
  Add2 : Sum  Inputs=|++  OutDataTypeStr=Inherit: Same as first input
  Data Type Conversion17 : DataTypeConversion  OutDataTypeStr=fixdt(1,11,10)  SaturateOnIntegerOverflow=off  RndMeth=Floor
  Delay : Delay  DelayLength=1
  Delay1 : Delay  DelayLength=1  InitialCondition=0
  Delay2 : Delay  InitialCondition=0
  Delay3 : Delay  InitialCondition=0
  Delay4 : Delay  DelayLength=1  InitialCondition=0
  Delay5 : Delay  InitialCondition=0
  Delay6 : Delay  DelayLength=1
  K1 : Gain  Gain=fi(config.SSLoopFilterPropGain,1,24,24)  ParamDataTypeStr=Inherit: Inherit from 'Gain'  OutDataTypeStr=Inherit: Same as input
  K2 : Gain  Gain=fi(config.SSLoopFilterIntegGain,1,24,24)  ParamDataTypeStr=Inherit: Inherit from 'Gain'  OutDataTypeStr=Inherit: Same as input
  v : Outport
  wires:
  Delay6/1 -> Add2/1
  K1/1 -> Delay3/1
  Add2/1 -> Delay4/1, Delay/1
  K2/1 -> Delay5/1
  Data Type Conversion17/1 -> v/1
  Delay2/1 -> K2/1, K1/1
  Delay4/1 -> Add/2
  Delay1/1 -> Add/1
  Add/1 -> Data Type Conversion17/1
  e/1 -> Delay2/1
  Delay3/1 -> Delay1/1
  Delay5/1 -> Delay6/1
  Delay/1 -> Add2/2

== system soc_dvbs2_fpga/DVBS2/DVBS2 TxRx/DVB-S2 HDL Receiver/Synchronizer and PL Header Decoder/Time Frequency and Coarse Phase Synchronizer/Time and Coarse Frequency Synchronizer/Symbol Synchronizer/Rate Handle ==
  dataIn : Inport
  strobe : Inport  Port=2
  validIn : Inport  Port=3
  Compare To Constant : simulink/Logic and Bit Operations/Compare To Constant  relop===  const=config.SamplesPerSymbol - 1  OutDataTypeStr=boolean
  Downsample : DownSample  N=config.SamplesPerSymbol  RateOptions=Allow multirate processing
  Downsample1 : DownSample  N=config.SamplesPerSymbol  RateOptions=Allow multirate processing
  FIFO : Subsystem
  HDL Counter : hdlsllib/Sources/HDL Counter  CountType=Count limited  CountInit=0  CountStep=1  CountMax=config.SamplesPerSymbol - 1  CountFromType=Initial value  CountFrom=0  CountResetPort=off  CountLoadPort=off  CountEnbPort=on  CountDirPort=off  CountHitOutputPort=off  CountDataType=Unsigned  CountWordLen=nextpow2(config.SamplesPerSymbol - 1)  CountFracLen=0  CountSampTime=1
  Logical Operator : Logic  AllPortsSameDT=off  OutDataTypeStr=boolean
  Unit Delay Enabled Synchronous : hdlsllib/Discrete/Unit Delay Enabled Synchronous  InitialCondition=0.0  SampleTime=-1
  monostable : MATLAB Function  TreatAsAtomicUnit=on  mask{nClocks=config.SamplesPerSymbol}
      mask prompts: nClocks "Number of Clocks:"
  dataOut : Outport
  validOut : Outport  Port=2
  wires:
  Unit Delay Enabled Synchronous/1 -> Downsample/1
  monostable/1(out) -> Downsample1/1
  FIFO/2(outValid) -> monostable/1(trigger), Unit Delay Enabled Synchronous/2
  FIFO/1(out) -> Unit Delay Enabled Synchronous/1
  Logical Operator/1 -> FIFO/3(pop)
  strobe/1 -> FIFO/2(push)
  dataIn/1 -> FIFO/1(data)
  validIn/1 -> Logical Operator/1, HDL Counter/1
  Downsample/1 -> dataOut/1
  Downsample1/1 -> validOut/1
  HDL Counter/1 -> Compare To Constant/1
  Compare To Constant/1 -> Logical Operator/2

== system soc_dvbs2_fpga/DVBS2/DVBS2 TxRx/DVB-S2 HDL Receiver/Demod Deinterleave and FECDecode/DVBS2 HDL Deinterleaver/RAM Address Generator/Generate and Add Read Base Address/No HDL Read Address Debug Scope/Wrap Address ==
  u : Inport
  Add : Sum  Inputs=+-  OutDataTypeStr=Inherit: Same as first input
  Compare To Constant : simulink/Logic and Bit Operations/Compare To Constant  relop=>=  const=ConfigRx.RAMCapacity  OutDataTypeStr=boolean
  Constant : Constant  Value=ConfigRx.RAMCapacity  OutDataTypeStr=Inherit: Inherit via back propagation  SampleTime=Tsamp
  Constant1 : Constant  Value=0  OutDataTypeStr=Inherit: Inherit via back propagation  SampleTime=Tsamp
  Data Type Duplicate : DataTypeDuplicate
  Data Type Duplicate1 : DataTypeDuplicate
  Data Type Conversion : DataTypeConversion  OutDataTypeStr=fixdt(0,nextpow2(ConfigRx.RAMCapacity),0)  SaturateOnIntegerOverflow=off  RndMeth=Floor
  Switch : Switch  Criteria=u2 ~= 0  SaturateOnIntegerOverflow=off  InputSameDT=off
  Switch1 : Switch  Criteria=u2 ~= 0  SaturateOnIntegerOverflow=off  InputSameDT=off
  y : Outport
  wires:
  Constant1/1 -> Switch1/3, Data Type Duplicate1/2
  Switch1/1 -> Add/2
  Data Type Conversion/1 -> y/1
  Constant/1 -> Data Type Duplicate/2, Data Type Duplicate1/1, Switch1/1
  Add/1 -> Switch/1
  Compare To Constant/1 -> Switch/2, Switch1/2
  Switch/1 -> Data Type Conversion/1
  u/1 -> Compare To Constant/1, Add/1, Data Type Duplicate/1, Switch/3

== system soc_dvbs2_fpga/DVBS2/DVBS2 TxRx/DVB-S2 HDL Receiver/Synchronizer and PL Header Decoder/PL Header Recovery/PL Header Decoder/ML Decoder/Get Min Index/For Each Subsystem ==
  valueIn : Inport  Partition=on  PartitionDimension=1  PartitionWidth=2  PartitionOffset=0
  idxIn : Inport  Port=2  Partition=on  PartitionDimension=1  PartitionWidth=2  PartitionOffset=0
  Delay{1..9} (9 alike) : Delay  DelayLength=1
  Demux : Demux  Outputs=2
  Demux1 : Demux  Outputs=2
  For Each : ForEach  DisableCoverage=on
  Relational Operator : RelationalOperator  Operator=<  OutDataTypeStr=boolean  RndMeth=Simplest  InputSameDT=off
  Switch : Switch  Criteria=u2 ~= 0  SaturateOnIntegerOverflow=off  InputSameDT=off
  Switch1 : Switch  Criteria=u2 ~= 0  SaturateOnIntegerOverflow=off  InputSameDT=off
  ValueOut : Outport  ConcatenationDimension=1
  idxOut : Outport  Port=2  ConcatenationDimension=1
  wires:
  Delay9/1 -> idxOut/1
  Delay8/1 -> ValueOut/1
  Delay7/1 -> Switch1/3
  Delay6/1 -> Switch1/1
  Delay5/1 -> Switch/3
  Delay4/1 -> Switch/1
  Delay2/1 -> Switch/2, Switch1/2
  Delay1/1 -> Demux1/1
  Delay3/1 -> Demux/1
  Switch/1 -> Delay8/1
  Relational Operator/1 -> Delay2/1
  Switch1/1 -> Delay9/1
  Demux1/2 -> Delay7/1
  Demux1/1 -> Delay6/1
  idxIn/1 -> Delay1/1
  Demux/2 -> Delay5/1, Relational Operator/2
  Demux/1 -> Delay4/1, Relational Operator/1
  valueIn/1 -> Delay3/1

== system soc_dvbs2_fpga/DVBS2/DVBS2 TxRx/DVB-S2 HDL Receiver/Synchronizer and PL Header Decoder/PL Header Recovery/PL Header Decoder/ML Decoder/Get Min Index/For Each Subsystem1 ==
  valueIn : Inport  Partition=on  PartitionDimension=1  PartitionWidth=2  PartitionOffset=0
  idxIn : Inport  Port=2  Partition=on  PartitionDimension=1  PartitionWidth=2  PartitionOffset=0
  Delay{1..9} (9 alike) : Delay  DelayLength=1
  Demux : Demux  Outputs=2
  Demux1 : Demux  Outputs=2
  For Each : ForEach  DisableCoverage=on
  Relational Operator : RelationalOperator  Operator=<  OutDataTypeStr=boolean  RndMeth=Simplest  InputSameDT=off
  Switch : Switch  Criteria=u2 ~= 0  SaturateOnIntegerOverflow=off  InputSameDT=off
  Switch1 : Switch  Criteria=u2 ~= 0  SaturateOnIntegerOverflow=off  InputSameDT=off
  ValueOut : Outport  ConcatenationDimension=1
  idxOut : Outport  Port=2  ConcatenationDimension=1
  wires:
  valueIn/1 -> Delay3/1
  Demux/1 -> Relational Operator/1, Delay4/1
  Demux/2 -> Relational Operator/2, Delay5/1
  idxIn/1 -> Delay1/1
  Demux1/1 -> Delay6/1
  Demux1/2 -> Delay7/1
  Switch1/1 -> Delay9/1
  Relational Operator/1 -> Delay2/1
  Switch/1 -> Delay8/1
  Delay3/1 -> Demux/1
  Delay1/1 -> Demux1/1
  Delay2/1 -> Switch1/2, Switch/2
  Delay4/1 -> Switch/1
  Delay5/1 -> Switch/3
  Delay6/1 -> Switch1/1
  Delay7/1 -> Switch1/3
  Delay8/1 -> ValueOut/1
  Delay9/1 -> idxOut/1

== system soc_dvbs2_fpga/DVBS2/DVBS2 TxRx/DVB-S2 HDL Receiver/Synchronizer and PL Header Decoder/PL Header Recovery/PL Header Decoder/ML Decoder/Get Min Index/For Each Subsystem2 ==
  valueIn : Inport  Partition=on  PartitionDimension=1  PartitionWidth=2  PartitionOffset=0
  idxIn : Inport  Port=2  Partition=on  PartitionDimension=1  PartitionWidth=2  PartitionOffset=0
  Delay{1..9} (9 alike) : Delay  DelayLength=1
  Demux : Demux  Outputs=2
  Demux1 : Demux  Outputs=2
  For Each : ForEach  DisableCoverage=on
  Relational Operator : RelationalOperator  Operator=<  OutDataTypeStr=boolean  RndMeth=Simplest  InputSameDT=off
  Switch : Switch  Criteria=u2 ~= 0  SaturateOnIntegerOverflow=off  InputSameDT=off
  Switch1 : Switch  Criteria=u2 ~= 0  SaturateOnIntegerOverflow=off  InputSameDT=off
  ValueOut : Outport  ConcatenationDimension=1
  idxOut : Outport  Port=2  ConcatenationDimension=1
  wires:
  Delay9/1 -> idxOut/1
  Delay8/1 -> ValueOut/1
  Delay7/1 -> Switch1/3
  Delay6/1 -> Switch1/1
  Delay5/1 -> Switch/3
  Delay4/1 -> Switch/1
  Delay2/1 -> Switch/2, Switch1/2
  Delay1/1 -> Demux1/1
  Delay3/1 -> Demux/1
  Switch/1 -> Delay8/1
  Relational Operator/1 -> Delay2/1
  Switch1/1 -> Delay9/1
  Demux1/2 -> Delay7/1
  Demux1/1 -> Delay6/1
  idxIn/1 -> Delay1/1
  Demux/2 -> Delay5/1, Relational Operator/2
  Demux/1 -> Delay4/1, Relational Operator/1
  valueIn/1 -> Delay3/1

== system soc_dvbs2_fpga/DVBS2/DVBS2 TxRx/DVB-S2 HDL Receiver/Synchronizer and PL Header Decoder/PL Header Recovery/PL Header Decoder/ML Decoder/Get Min Index/For Each Subsystem3 ==
  valueIn : Inport  Partition=on  PartitionDimension=1  PartitionWidth=2  PartitionOffset=0
  idxIn : Inport  Port=2  Partition=on  PartitionDimension=1  PartitionWidth=2  PartitionOffset=0
  Delay{1..9} (9 alike) : Delay  DelayLength=1
  Demux : Demux  Outputs=2
  Demux1 : Demux  Outputs=2
  For Each : ForEach  DisableCoverage=on
  Relational Operator : RelationalOperator  Operator=<  OutDataTypeStr=boolean  RndMeth=Simplest  InputSameDT=off
  Switch : Switch  Criteria=u2 ~= 0  SaturateOnIntegerOverflow=off  InputSameDT=off
  Switch1 : Switch  Criteria=u2 ~= 0  SaturateOnIntegerOverflow=off  InputSameDT=off
  ValueOut : Outport  ConcatenationDimension=1
  idxOut : Outport  Port=2  ConcatenationDimension=1
  wires:
  valueIn/1 -> Delay3/1
  Demux/1 -> Relational Operator/1, Delay4/1
  Demux/2 -> Relational Operator/2, Delay5/1
  idxIn/1 -> Delay1/1
  Demux1/1 -> Delay6/1
  Demux1/2 -> Delay7/1
  Switch1/1 -> Delay9/1
  Relational Operator/1 -> Delay2/1
  Switch/1 -> Delay8/1
  Delay3/1 -> Demux/1
  Delay1/1 -> Demux1/1
  Delay2/1 -> Switch1/2, Switch/2
  Delay4/1 -> Switch/1
  Delay5/1 -> Switch/3
  Delay6/1 -> Switch1/1
  Delay7/1 -> Switch1/3
  Delay8/1 -> ValueOut/1
  Delay9/1 -> idxOut/1

== system soc_dvbs2_fpga/DVBS2/DVBS2 TxRx/DVB-S2 HDL Receiver/Synchronizer and PL Header Decoder/PL Header Recovery/PL Header Decoder/ML Decoder/Get Min Index/For Each Subsystem4 ==
  valueIn : Inport  Partition=on  PartitionDimension=1  PartitionWidth=2  PartitionOffset=0
  idxIn : Inport  Port=2  Partition=on  PartitionDimension=1  PartitionWidth=2  PartitionOffset=0
  Delay{1..9} (9 alike) : Delay  DelayLength=1
  Demux : Demux  Outputs=2
  Demux1 : Demux  Outputs=2
  For Each : ForEach  DisableCoverage=on
  Relational Operator : RelationalOperator  Operator=<  OutDataTypeStr=boolean  RndMeth=Simplest  InputSameDT=off
  Switch : Switch  Criteria=u2 ~= 0  SaturateOnIntegerOverflow=off  InputSameDT=off
  Switch1 : Switch  Criteria=u2 ~= 0  SaturateOnIntegerOverflow=off  InputSameDT=off
  ValueOut : Outport  ConcatenationDimension=1
  idxOut : Outport  Port=2  ConcatenationDimension=1
  wires:
  Delay9/1 -> idxOut/1
  Delay8/1 -> ValueOut/1
  Delay7/1 -> Switch1/3
  Delay6/1 -> Switch1/1
  Delay5/1 -> Switch/3
  Delay4/1 -> Switch/1
  Delay2/1 -> Switch/2, Switch1/2
  Delay1/1 -> Demux1/1
  Delay3/1 -> Demux/1
  Switch/1 -> Delay8/1
  Relational Operator/1 -> Delay2/1
  Switch1/1 -> Delay9/1
  Demux1/2 -> Delay7/1
  Demux1/1 -> Delay6/1
  idxIn/1 -> Delay1/1
  Demux/2 -> Delay5/1, Relational Operator/2
  Demux/1 -> Delay4/1, Relational Operator/1
  valueIn/1 -> Delay3/1

== system soc_dvbs2_fpga/DVBS2/DVBS2 TxRx/DVB-S2 HDL Receiver/Synchronizer and PL Header Decoder/PL Header Recovery/PL Header Decoder/ML Decoder/Get Min Index/For Each Subsystem5 ==
  valueIn : Inport
  idxIn : Inport  Port=2
  Delay{1..6} (6 alike) : Delay  DelayLength=1
  Demux : Demux  Outputs=2
  Demux1 : Demux  Outputs=2
  Relational Operator : RelationalOperator  Operator=<  OutDataTypeStr=boolean  RndMeth=Simplest  InputSameDT=off
  Switch1 : Switch  Criteria=u2 ~= 0  SaturateOnIntegerOverflow=off  InputSameDT=off
  idxOut : Outport
  wires:
  Delay6/1 -> idxOut/1
  Delay5/1 -> Switch1/3
  Delay4/1 -> Switch1/2
  Delay2/1 -> Switch1/1
  Delay1/1 -> Demux1/1
  Delay3/1 -> Demux/1
  valueIn/1 -> Delay3/1
  Demux/1 -> Relational Operator/1
  Demux/2 -> Relational Operator/2
  idxIn/1 -> Delay1/1
  Demux1/1 -> Delay2/1
  Demux1/2 -> Delay5/1
  Switch1/1 -> Delay6/1
  Relational Operator/1 -> Delay4/1

== system soc_dvbs2_fpga/DVBS2/DVBS2 TxRx/DVB-S2 HDL Receiver/Synchronizer and PL Header Decoder/PL Header Recovery/PL Header Decoder/ML Decoder/Integer to Bit Convertor/For Each Subsystem ==
  In1 : Inport  Partition=on  PartitionDimension=1  PartitionWidth=1  PartitionOffset=0
  Extract Bits2 : simulink/Logic and Bit Operations/Extract Bits  bitsToExtract=Upper half  numBits=8  bitIdxRange=[32 63]  outScalingMode=Treat bit field as an integer
  Extract Bits3 : simulink/Logic and Bit Operations/Extract Bits  bitsToExtract=Lower half  numBits=8  bitIdxRange=[32 63]  outScalingMode=Treat bit field as an integer
  For Each : ForEach  DisableCoverage=on
  Mux1 : Mux  Inputs=2
  Out1 : Outport  ConcatenationDimension=1
  wires:
  Extract Bits3/1 -> Mux1/2
  In1/1 -> Extract Bits2/1, Extract Bits3/1
  Extract Bits2/1 -> Mux1/1
  Mux1/1 -> Out1/1

== system soc_dvbs2_fpga/DVBS2/DVBS2 TxRx/DVB-S2 HDL Receiver/Synchronizer and PL Header Decoder/PL Header Recovery/PL Header Decoder/ML Decoder/Integer to Bit Convertor/For Each Subsystem1 ==
  In1 : Inport  Partition=on  PartitionDimension=1  PartitionWidth=1  PartitionOffset=0
  Extract Bits2 : simulink/Logic and Bit Operations/Extract Bits  bitsToExtract=Upper half  numBits=8  bitIdxRange=[32 63]  outScalingMode=Treat bit field as an integer
  Extract Bits3 : simulink/Logic and Bit Operations/Extract Bits  bitsToExtract=Lower half  numBits=8  bitIdxRange=[32 63]  outScalingMode=Treat bit field as an integer
  For Each : ForEach  DisableCoverage=on
  Mux1 : Mux  Inputs=2
  Out1 : Outport  ConcatenationDimension=1
  wires:
  Mux1/1 -> Out1/1
  Extract Bits2/1 -> Mux1/1
  In1/1 -> Extract Bits3/1, Extract Bits2/1
  Extract Bits3/1 -> Mux1/2

== system soc_dvbs2_fpga/DVBS2/DVBS2 TxRx/DVB-S2 HDL Receiver/Synchronizer and PL Header Decoder/PL Header Recovery/PL Header Decoder/ML Decoder/Integer to Bit Convertor/For Each Subsystem2 ==
  In1 : Inport  Partition=on  PartitionDimension=1  PartitionWidth=1  PartitionOffset=0
  Extract Bits2 : simulink/Logic and Bit Operations/Extract Bits  bitsToExtract=Upper half  numBits=8  bitIdxRange=[32 63]  outScalingMode=Treat bit field as an integer
  Extract Bits3 : simulink/Logic and Bit Operations/Extract Bits  bitsToExtract=Lower half  numBits=8  bitIdxRange=[32 63]  outScalingMode=Treat bit field as an integer
  For Each : ForEach  DisableCoverage=on
  Mux1 : Mux  Inputs=2
  Out1 : Outport  ConcatenationDimension=1
  wires:
  Extract Bits3/1 -> Mux1/2
  In1/1 -> Extract Bits2/1, Extract Bits3/1
  Extract Bits2/1 -> Mux1/1
  Mux1/1 -> Out1/1

== system soc_dvbs2_fpga/DVBS2/DVBS2 TxRx/DVB-S2 HDL Receiver/Synchronizer and PL Header Decoder/PL Header Recovery/PL Header Decoder/ML Decoder/Integer to Bit Convertor/For Each Subsystem3 ==
  In1 : Inport  Partition=on  PartitionDimension=1  PartitionWidth=1  PartitionOffset=0
  Extract Bits2 : simulink/Logic and Bit Operations/Extract Bits  bitsToExtract=Upper half  numBits=8  bitIdxRange=[32 63]  outScalingMode=Treat bit field as an integer
  Extract Bits3 : simulink/Logic and Bit Operations/Extract Bits  bitsToExtract=Lower half  numBits=8  bitIdxRange=[32 63]  outScalingMode=Treat bit field as an integer
  For Each : ForEach  DisableCoverage=on
  Mux1 : Mux  Inputs=2
  Out1 : Outport  ConcatenationDimension=1
  wires:
  Mux1/1 -> Out1/1
  Extract Bits2/1 -> Mux1/1
  In1/1 -> Extract Bits3/1, Extract Bits2/1
  Extract Bits3/1 -> Mux1/2

== system soc_dvbs2_fpga/DVBS2/DVBS2 TxRx/DVB-S2 HDL Receiver/Synchronizer and PL Header Decoder/PL Header Recovery/PL Header Decoder/ML Decoder/Integer to Bit Convertor/For Each Subsystem4 ==
  In1 : Inport  Partition=on  PartitionDimension=1  PartitionWidth=1  PartitionOffset=0
  Extract Bits2 : simulink/Logic and Bit Operations/Extract Bits  bitsToExtract=Upper half  numBits=8  bitIdxRange=[32 63]  outScalingMode=Treat bit field as an integer
  Extract Bits3 : simulink/Logic and Bit Operations/Extract Bits  bitsToExtract=Lower half  numBits=8  bitIdxRange=[32 63]  outScalingMode=Treat bit field as an integer
  For Each : ForEach  DisableCoverage=on
  Mux1 : Mux  Inputs=2
  Out1 : Outport  ConcatenationDimension=1
  wires:
  Mux1/1 -> Out1/1
  Extract Bits2/1 -> Mux1/1
  In1/1 -> Extract Bits3/1, Extract Bits2/1
  Extract Bits3/1 -> Mux1/2

== system soc_dvbs2_fpga/DVBS2/DVBS2 TxRx/DVB-S2 HDL Receiver/Synchronizer and PL Header Decoder/PL Header Recovery/PL Header Decoder/ML Decoder/Integer to Bit Convertor/For Each Subsystem5 ==
  In1 : Inport  Partition=on  PartitionDimension=1  PartitionWidth=1  PartitionOffset=0
  Extract Bits2 : simulink/Logic and Bit Operations/Extract Bits  bitsToExtract=Upper half  numBits=8  bitIdxRange=[32 63]  outScalingMode=Treat bit field as an integer
  Extract Bits3 : simulink/Logic and Bit Operations/Extract Bits  bitsToExtract=Lower half  numBits=8  bitIdxRange=[32 63]  outScalingMode=Treat bit field as an integer
  For Each : ForEach  DisableCoverage=on
  Mux1 : Mux  Inputs=2
  Out1 : Outport  ConcatenationDimension=1
  wires:
  Extract Bits3/1 -> Mux1/2
  In1/1 -> Extract Bits2/1, Extract Bits3/1
  Extract Bits2/1 -> Mux1/1
  Mux1/1 -> Out1/1

== system soc_dvbs2_fpga/DVBS2/DVBS2 TxRx/DVB-S2 HDL Receiver/Synchronizer and PL Header Decoder/PL Header Recovery/PL Header Decoder/ML Decoder/Integer to Bit Convertor/For Each Subsystem6 ==
  In1 : Inport  Partition=on  PartitionDimension=1  PartitionWidth=1  PartitionOffset=0
  Extract Bits2 : simulink/Logic and Bit Operations/Extract Bits  bitsToExtract=Upper half  numBits=8  bitIdxRange=[32 63]  outScalingMode=Treat bit field as an integer
  Extract Bits3 : simulink/Logic and Bit Operations/Extract Bits  bitsToExtract=Lower half  numBits=8  bitIdxRange=[32 63]  outScalingMode=Treat bit field as an integer
  For Each : ForEach  DisableCoverage=on
  Mux1 : Mux  Inputs=2
  Out1 : Outport  ConcatenationDimension=1
  wires:
  Mux1/1 -> Out1/1
  Extract Bits2/1 -> Mux1/1
  In1/1 -> Extract Bits3/1, Extract Bits2/1
  Extract Bits3/1 -> Mux1/2

== system soc_dvbs2_fpga/DVBS2/DVBS2 TxRx/DVB-S2 HDL Receiver/Synchronizer and PL Header Decoder/PL Header Recovery/PL Header Decoder/ML Decoder/Integer to Bit Convertor/For Each Subsystem7 ==
  In1 : Inport  Partition=on  PartitionDimension=1  PartitionWidth=1  PartitionOffset=0
  Extract Bits2 : simulink/Logic and Bit Operations/Extract Bits  bitsToExtract=Upper half  numBits=8  bitIdxRange=[32 63]  outScalingMode=Treat bit field as an integer
  Extract Bits3 : simulink/Logic and Bit Operations/Extract Bits  bitsToExtract=Lower half  numBits=8  bitIdxRange=[32 63]  outScalingMode=Treat bit field as an integer
  For Each : ForEach  DisableCoverage=on
  Mux1 : Mux  Inputs=2
  Out1 : Outport  ConcatenationDimension=1
  wires:
  Extract Bits3/1 -> Mux1/2
  In1/1 -> Extract Bits2/1, Extract Bits3/1
  Extract Bits2/1 -> Mux1/1
  Mux1/1 -> Out1/1

== system soc_dvbs2_fpga/DVBS2/DVBS2 TxRx/DVB-S2 HDL Receiver/Synchronizer and PL Header Decoder/PL Header Recovery/PL Header Decoder/ML Decoder/Integer to Bit Convertor/Subsystem ==
  u : Inport
  u1 : Inport  Port=2
  Extract Bits2 : simulink/Logic and Bit Operations/Extract Bits  bitsToExtract=Upper half  numBits=8  bitIdxRange=[32 63]  outScalingMode=Treat bit field as an integer
  Extract Bits3 : simulink/Logic and Bit Operations/Extract Bits  bitsToExtract=Lower half  numBits=8  bitIdxRange=[32 63]  outScalingMode=Treat bit field as an integer
  Mux1 : Mux  Inputs=2
  Out1 : Outport
  wires:
  Mux1/1 -> Out1/1
  u1/1 -> Extract Bits3/1
  u/1 -> Extract Bits2/1
  Extract Bits3/1 -> Mux1/2
  Extract Bits2/1 -> Mux1/1

== system soc_dvbs2_fpga/DVBS2/DVBS2 TxRx/DVB-S2 HDL Receiver/Synchronizer and PL Header Decoder/PL Header Recovery/PL Header Decoder/ML Decoder/Integer to Bit Convertor/Subsystem1 ==
  u : Inport
  u1 : Inport  Port=2
  Extract Bits2 : simulink/Logic and Bit Operations/Extract Bits  bitsToExtract=Upper half  numBits=8  bitIdxRange=[32 63]  outScalingMode=Treat bit field as an integer
  Extract Bits3 : simulink/Logic and Bit Operations/Extract Bits  bitsToExtract=Lower half  numBits=8  bitIdxRange=[32 63]  outScalingMode=Treat bit field as an integer
  Mux1 : Mux  Inputs=2
  Out1 : Outport
  wires:
  Extract Bits2/1 -> Mux1/1
  Extract Bits3/1 -> Mux1/2
  u/1 -> Extract Bits2/1
  u1/1 -> Extract Bits3/1
  Mux1/1 -> Out1/1
